simulink model "untitled"  (R2020a)
settings: Solver=VariableStepAuto  StartTime=0.0  StopTime=10.0  RelTol=1e-3
libraries: fuzblock x1
settings Model: Creator=Asus  LastModifiedBy=Asus

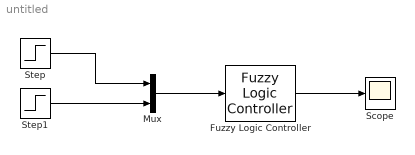
== system untitled ==
  Fuzzy Logic Controller : fuzblock/Fuzzy Logic  Controller  FIS='FIS7.fis'  OutputSampleNumber=101  DataType=double  FuzzifiedInputs=off  RuleFiringStrengths=off  RuleOutputs=off  AggregatedOutputs=off  SimulateUsing=Interpreted execution  OutOfRangeInputValueMessage=warning  NoRuleFiredMessage=warning  EmptyOutputFuzzySetMessage=warning
  Mux : Mux  Inputs=2
  Scope : Scope
  Step : Step  After=24  SampleTime=0
  Step1 : Step  After=80  SampleTime=0
  wires:
  Mux/1 -> Fuzzy Logic Controller/1
  Fuzzy Logic Controller/1 -> Scope/1
  Step/1 -> Mux/1
  Step1/1 -> Mux/2
